simulink model "dbx_control_v0_01"  (R2015a)
settings: Solver=FixedStepDiscrete  SolverMode=SingleTasking  StartTime=0.0  StopTime=10.0  FixedStep=T_ctrl  RelTol=1e-3
values from neighbouring files (symbols this model uses):
  delta_ail_Asim_0 = 0    [FW_init.m]    (also in simple_all.m = single(delta_ail_Asim_0))
  delta_rv_sim_0 = deg2rad(0)    [FW_init.m]    (also in simple_all.m = single(delta_rv_sim_0))
  Euler_0 = zeros(3,1)    [FW_init.m]    (also in simple_all.m = single(Euler_0))
  Euler_0_2 = Euler_0(2)    [FW_init.m]
  FCS_control_mix = inv(B_adim)    [FCS_fw_params.m]
  Flaps_ang_deg = 0    [FCS_fw_params.m]    (also in simple_all.m = single(Flaps_ang_deg))
  Kd_h = 0.05    [FCS_fw_params.m]
  Ki_h = 0.05    [FCS_fw_params.m]
  Ki_p = 0    [FCS_fw_params.m]
  Ki_phi = 0.5    [FCS_fw_params.m]
  Ki_q = 0.01    [FCS_fw_params.m]
  Ki_theta = 0.1    [FCS_fw_params.m]
  Ki_u = 0.03    [FCS_fw_params.m]
  Kp_h = 0.1    [FCS_fw_params.m]
  Kp_p = 0.01    [FCS_fw_params.m]
  Kp_phi = 10    [FCS_fw_params.m]
  Kp_q = 0.07    [FCS_fw_params.m]
  Kp_theta = 3    [FCS_fw_params.m]
  Kp_u = 0.1    [FCS_fw_params.m]
  m = m_OE + m_PL    (= 14.5)    [SetupComplete.m]    (also in simple_all.m = single(m))
  S_w = 0.75    [SetupComplete.m]    (also in simple_all.m = single(S_w))
  T_ctrl = 0.01    [Run_DBX.m]    (also in simple_all.m = double(T_ctrl))
  tau_1_0 = 0.5    [FW_init.m]    (also in simple_all.m = single(tau_1_0))
undefined symbols (not defined in the file or in its folder): Servo_calib
libraries: DBX_model x28, simulink x3
settings Model: ExtModeTrigDuration=5000  TunableVars=Flaps_ang_deg,Kd_h,Ki_h,Ki_p,Ki_phi,Ki_q,Ki_theta,Ki_u,Kp_h,Kp_p,Kp_phi,Kp_q,Kp_theta,Kp_u  TunableVarsStorageClass=Auto,Auto,Auto,Auto,Auto,Auto,Auto,Auto,Auto,Auto,Auto,Auto,Auto,Auto  TunableVarsTypeQualifier=,,,,,,,,,,,,,  Creator=DavidTorres  LastModifiedBy=David
settings DataIOCC: LimitDataPoints=off  SaveOutput=off  SignalLogging=off  DSMLogging=off  VisualizeSimOutput=off  SaveTime=off
settings OptimizationCC: InlineParams=on  UseDivisionForNetSlopeComputation=on  UseSpecifiedMinMax=on  EfficientFloat2IntCast=on  OptimizeModelRefInitCode=on  MaxStackSize=64  SimCompilerOptimization=on
settings DebuggingCC: SaveWithParameterizedLinksMsg=none  IntegerOverflowMsg=error  StrictBusMsg=ErrorOnBusTreatedAsVector  IntegerSaturationMsg=error
settings HardwareCC: ProdLargestAtomicInteger=Long  ProdLargestAtomicFloat=Double  ProdEndianess=LittleEndian  ProdHWDeviceType=ARM Compatible->ARM Cortex  TargetLongLongMode=on  TargetIntDivRoundTo=Zero  TargetEndianess=LittleEndian  TargetHWDeviceType=MATLAB Host  ProdEqTarget=off
settings ModelReferenceCC: ModelReferenceNumInstancesAllowed=Single  ModelReferencePassRootInputsByReference=off
settings RTWCC: SystemTargetFile=ert.tlc  GenCodeOnly=on  TemplateMakefile=ert_default_tmf  Description=Embedded Coder  BuildConfiguration=Faster Runs
settings CodeAppCC: IgnoreCustomStorageClasses=off
settings ERTTargetCC: GenerateSampleERTMain=off  ParMdlRefBuildCompliant=on  CompOptLevelCompliant=on  ConcurrentExecutionCompliant=on  ERTFirstTimeCompliant=on  SupportNonFinite=off  SupportComplex=off  SupportContinuousTime=off  SupportVariableSizeSignals=off  ModelStepFunctionPrototypeControlCompliant=on  CPPClassGenCompliant=on  InlinedParameterPlacement=Hierarchical  ERTCustomFileTemplate=example_file_process.tlc

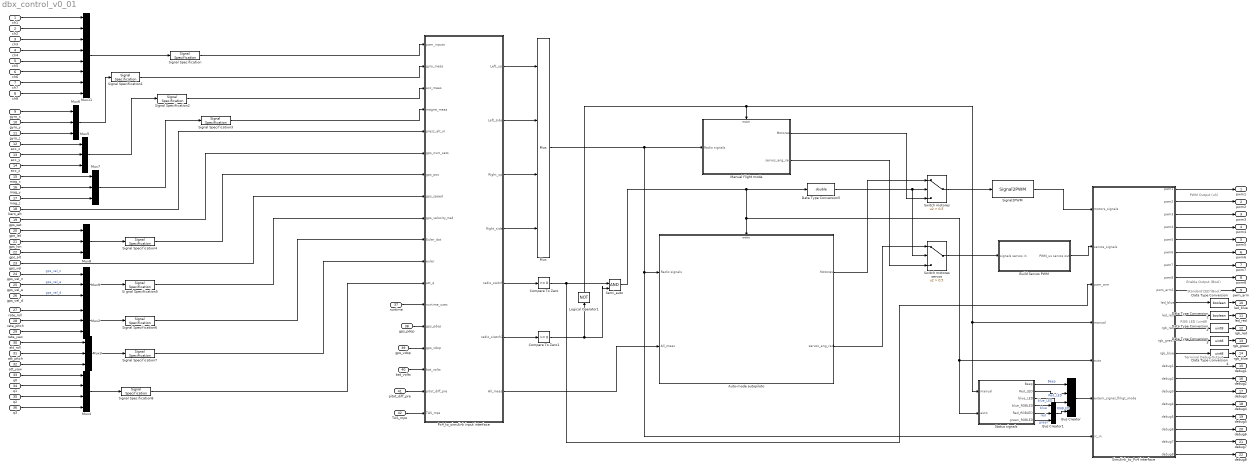
== system dbx_control_v0_01 ==
  note: Terminal Debug Output
  note: RGB LED (uint8)
  note: Standard LED (Bool)
  note: PWM Output (uS)
  note: Enable Output (Bool)
  ch1 : Inport  PortDimensions=[1,1]  SampleTime=T_ctrl
  ch2 : Inport  Port=2  PortDimensions=[1,1]  SampleTime=T_ctrl
  ch3 : Inport  Port=3  PortDimensions=[1,1]  SampleTime=T_ctrl
  ch4 : Inport  Port=4  PortDimensions=[1,1]  SampleTime=T_ctrl
  ch5 : Inport  Port=5  PortDimensions=[1,1]  SampleTime=T_ctrl
  ch6 : Inport  Port=6  PortDimensions=[1,1]  SampleTime=T_ctrl
  ch7 : Inport  Port=7  PortDimensions=[1,1]  SampleTime=T_ctrl
  ch8 : Inport  Port=8  PortDimensions=[1,1]  SampleTime=T_ctrl
  gyro_x : Inport  Port=9  PortDimensions=[1,1]  SampleTime=T_ctrl
  gyro_y : Inport  Port=10  PortDimensions=[1,1]  SampleTime=T_ctrl
  gyro_z : Inport  Port=11  PortDimensions=[1,1]  SampleTime=T_ctrl
  acc_x : Inport  Port=12  PortDimensions=[1,1]  SampleTime=T_ctrl
  acc_y : Inport  Port=13  PortDimensions=[1,1]  SampleTime=T_ctrl
  acc_z : Inport  Port=14  PortDimensions=[1,1]  SampleTime=T_ctrl
  mag_x : Inport  Port=15  PortDimensions=[1,1]  SampleTime=T_ctrl
  mag_y : Inport  Port=16  PortDimensions=[1,1]  SampleTime=T_ctrl
  mag_z : Inport  Port=17  PortDimensions=[1,1]  SampleTime=T_ctrl
  baro_alt : Inport  Port=18  PortDimensions=[1,1]  SampleTime=T_ctrl
  gps_sat : Inport  Port=19  PortDimensions=[1,1]  SampleTime=T_ctrl
  gps_lat : Inport  Port=20  PortDimensions=[1,1]  SampleTime=T_ctrl
  gps_lon : Inport  Port=21  PortDimensions=[1,1]  SampleTime=T_ctrl
  gps_alt : Inport  Port=22  PortDimensions=[1,1]  SampleTime=T_ctrl
  gps_vel : Inport  Port=23  PortDimensions=[1,1]  SampleTime=T_ctrl
  gps_vel_n : Inport  Port=24  PortDimensions=[1,1]  SampleTime=T_ctrl
  gps_vel_e : Inport  Port=25  PortDimensions=[1,1]  SampleTime=T_ctrl
  gps_vel_d : Inport  Port=26  PortDimensions=[1,1]  SampleTime=T_ctrl
  rate_roll : Inport  Port=27  PortDimensions=[1,1]  SampleTime=T_ctrl
  rate_pitch : Inport  Port=28  PortDimensions=[1,1]  SampleTime=T_ctrl
  rate_yaw : Inport  Port=29  PortDimensions=[1,1]  SampleTime=T_ctrl
  att_roll : Inport  Port=30  PortDimensions=[1,1]  SampleTime=T_ctrl
  att_pitch : Inport  Port=31  PortDimensions=[1,1]  SampleTime=T_ctrl
  att_yaw : Inport  Port=32  PortDimensions=[1,1]  SampleTime=T_ctrl
  q0 : Inport  Port=33  PortDimensions=[1,1]  SampleTime=T_ctrl
  q1 : Inport  Port=34  PortDimensions=[1,1]  SampleTime=T_ctrl
  q2 : Inport  Port=35  PortDimensions=[1,1]  SampleTime=T_ctrl
  q3 : Inport  Port=36  PortDimensions=[1,1]  SampleTime=T_ctrl
  runtime : Inport  Port=37  PortDimensions=[1,1]  SampleTime=T_ctrl
  gps_pdop : Inport  Port=38  PortDimensions=[1,1]  SampleTime=T_ctrl
  gps_vdop : Inport  Port=39  PortDimensions=[1,1]  SampleTime=T_ctrl
  bat_volts : Inport  Port=40  PortDimensions=[1,1]  SampleTime=T_ctrl
  pitot_diff_pre : Inport  Port=41  SampleTime=0.01
  TAS_mps : Inport  Port=42  SampleTime=0.01
  Auto-mode autopiloto : Subsystem  TreatAsAtomicUnit=on
  Build Servos PWM : Subsystem  TreatAsAtomicUnit=on
  Bus Creator : BusCreator
  Bus Creator1 : BusCreator  Inputs=3
  Compare To Zero : simulink/Logic and Bit Operations/Compare To Zero  relop=>=  OutDataTypeStr=boolean
  Compare To Zero1 : simulink/Logic and Bit Operations/Compare To Zero  relop=>=  OutDataTypeStr=boolean
  Data Type Conversion : DataTypeConversion  OutDataTypeStr=boolean
  Data Type Conversion1 : DataTypeConversion  OutDataTypeStr=boolean
  Data Type Conversion2 : DataTypeConversion  OutDataTypeStr=uint8
  Data Type Conversion3 : DataTypeConversion  OutDataTypeStr=uint8
  Data Type Conversion4 : DataTypeConversion  OutDataTypeStr=uint8
  Data Type Conversion5 : DataTypeConversion  OutDataTypeStr=double
  Logical Operator1 : Logic  Operator=NOT  IconShape=distinctive  AllPortsSameDT=off  OutDataTypeStr=boolean
  Manual flight mode : Subsystem  TreatAsAtomicUnit=on
  Mux : Mux
  Mux11 : Mux  Inputs=8
  Mux{2..3,5..9} (7 alike) : Mux  Inputs=3
  Mux4 : Mux
  Px4_to_simulink input interface : Subsystem
  Semi_auto : Logic  IconShape=distinctive  AllPortsSameDT=off  OutDataTypeStr=boolean
  Si gnal Specification5 : SignalSpecification  Dimensions=[3,1]
  Signal Specification : SignalSpecification  Dimensions=[8,1]
  Signal Specification{1..4,6..7} (6 alike) : SignalSpecification  Dimensions=[3,1]
  Signal Specification8 : SignalSpecification  Dimensions=[4,1]
  Signal2PWM : DBX_model/Signal2PWM  b=1  d=0  a=1900  c=1100
  Simulink_to_Px4 interface : Subsystem
  Status signals : Subsystem  TreatAsAtomicUnit=on
  Switch motores : Switch  Criteria=u2 > Threshold  Threshold=0.5
  Switch motores servos : Switch  Criteria=u2 > Threshold  Threshold=0.5
  pwm1 : Outport  PortDimensions=[1,1]
  pwm2 : Outport  Port=2  PortDimensions=[1,1]
  pwm3 : Outport  Port=3  PortDimensions=[1,1]
  pwm4 : Outport  Port=4  PortDimensions=[1,1]
  pwm5 : Outport  Port=5  PortDimensions=[1,1]
  pwm6 : Outport  Port=6  PortDimensions=[1,1]
  pwm7 : Outport  Port=7  PortDimensions=[1,1]
  pwm8 : Outport  Port=8  PortDimensions=[1,1]
  pwm_arm : Outport  Port=9  PortDimensions=[1,1]
  led_blue : Outport  Port=10  OutDataTypeStr=boolean  PortDimensions=[1,1]
  led_red : Outport  Port=11  OutDataTypeStr=boolean  PortDimensions=[1,1]
  rgb_red : Outport  Port=12  OutDataTypeStr=uint8  PortDimensions=[1,1]
  rgb_green : Outport  Port=13  OutDataTypeStr=uint8  PortDimensions=[1,1]
  rgb_blue : Outport  Port=14  OutDataTypeStr=uint8  PortDimensions=[1,1]
  debug1 : Outport  Port=15  PortDimensions=[1,1]
  debug2 : Outport  Port=16  PortDimensions=[1,1]
  debug3 : Outport  Port=17  PortDimensions=[1,1]
  debug4 : Outport  Port=18  PortDimensions=[1,1]
  debug5 : Outport  Port=19  PortDimensions=[1,1]
  debug6 : Outport  Port=20  PortDimensions=[1,1]
  debug7 : Outport  Port=21  PortDimensions=[1,1]
  debug8 : Outport  Port=22  PortDimensions=[1,1]
  wires:
  Switch motores/1 -> Signal2PWM/1
  Switch motores servos/1 -> Build Servos PWM/1(signals servos in)
  Status signals/1(Beep) -> Bus Creator/1  "Beep"
  Status signals/2(Red_LED) -> Bus Creator/2  "Red_LED"
  Status signals/3(blue_LED) -> Bus Creator/3  "blue_LED"
  Status signals/4(blue_RGBLED) -> Bus Creator1/1  "blue"
  Status signals/5(Red_RGBLED) -> Bus Creator1/2  "red"
  Status signals/6(green_RGBLED) -> Bus Creator1/3  "green"
  Bus Creator1/1 -> Bus Creator/4  "RGBLED"
  Simulink_to_Px4 interface/1(pwm1) -> pwm1/1
  Simulink_to_Px4 interface/2(pwm2) -> pwm2/1
  Simulink_to_Px4 interface/3(pwm3) -> pwm3/1
  Simulink_to_Px4 interface/4(pwm4) -> pwm4/1
  Simulink_to_Px4 interface/5(pwm5) -> pwm5/1
  Simulink_to_Px4 interface/6(pwm6) -> pwm6/1
  Simulink_to_Px4 interface/7(pwm7) -> pwm7/1
  Simulink_to_Px4 interface/8(pwm8) -> pwm8/1
  Simulink_to_Px4 interface/10(led_blue) -> Data Type Conversion/1
  Simulink_to_Px4 interface/11(led_red) -> Data Type Conversion1/1
  Simulink_to_Px4 interface/15(debug1) -> debug1/1
  Simulink_to_Px4 interface/17(debug3) -> debug3/1
  Simulink_to_Px4 interface/18(debug4) -> debug4/1
  Simulink_to_Px4 interface/9(pwm_arm1) -> pwm_arm/1
  Simulink_to_Px4 interface/12(rgb_red) -> Data Type Conversion2/1
  Simulink_to_Px4 interface/13(rgb_green) -> Data Type Conversion3/1
  Simulink_to_Px4 interface/14(rgb_blue) -> Data Type Conversion4/1
  Simulink_to_Px4 interface/20(debug6) -> debug6/1
  Simulink_to_Px4 interface/21(debug7) -> debug7/1
  Simulink_to_Px4 interface/22(debug8) -> debug8/1
  Simulink_to_Px4 interface/19(debug5) -> debug5/1
  Data Type Conversion/1 -> led_blue/1
  Data Type Conversion1/1 -> led_red/1
  Data Type Conversion2/1 -> rgb_red/1
  Data Type Conversion3/1 -> rgb_green/1
  Data Type Conversion4/1 -> rgb_blue/1
  Simulink_to_Px4 interface/16(debug2) -> debug2/1
  Signal2PWM/1 -> Simulink_to_Px4 interface/1(motors_signals)
  Build Servos PWM/1(PWM_us servos out) -> Simulink_to_Px4 interface/2(servos_signals)
  Bus Creator/1 -> Simulink_to_Px4 interface/6(extern_signal_flihgt_mode)
  baro_alt/1 -> Px4_to_simulink input interface/5(press_alt_m)
  gyro_z/1 -> Mux6/3
  gyro_y/1 -> Mux6/2
  gyro_x/1 -> Mux6/1
  acc_z/1 -> Mux5/3
  acc_y/1 -> Mux5/2
  acc_x/1 -> Mux5/1
  mag_x/1 -> Mux7/1
  mag_y/1 -> Mux7/2
  mag_z/1 -> Mux7/3
  ch1/1 -> Mux11/1
  ch2/1 -> Mux11/2
  ch3/1 -> Mux11/3
  ch4/1 -> Mux11/4
  ch5/1 -> Mux11/5
  ch6/1 -> Mux11/6
  runtime/1 -> Px4_to_simulink input interface/13(runtime_usec)
  ch7/1 -> Mux11/7
  ch8/1 -> Mux11/8
  att_roll/1 -> Mux3/1
  att_pitch/1 -> Mux3/2
  att_yaw/1 -> Mux3/3
  q0/1 -> Mux4/1
  q1/1 -> Mux4/2
  q2/1 -> Mux4/3
  q3/1 -> Mux4/4
  rate_roll/1 -> Mux2/1
  rate_pitch/1 -> Mux2/2
  rate_yaw/1 -> Mux2/3
  gps_vel_n/1 -> Mux9/1  "gps_vel_n"
  gps_vel_e/1 -> Mux9/2  "gps_vel_e"
  gps_vel_d/1 -> Mux9/3  "gps_vel_d"
  gps_lat/1 -> Mux8/1
  gps_lon/1 -> Mux8/2
  gps_alt/1 -> Mux8/3
  gps_vel/1 -> Px4_to_simulink input interface/8(gps_speed)
  gps_sat/1 -> Px4_to_simulink input interface/6(gps_num_sats)
  Mux2/1 -> Signal Specification6/1
  Mux3/1 -> Signal Specification7/1
  Mux4/1 -> Signal Specification8/1
  Mux5/1 -> Signal Specification2/1
  Mux6/1 -> Signal Specification1/1
  Mux8/1 -> Signal Specification4/1
  Mux7/1 -> Signal Specification3/1
  Mux11/1 -> Signal Specification/1
  Mux9/1 -> Si gnal Specification5/1
  gps_pdop/1 -> Px4_to_simulink input interface/14(gps_pdop)
  gps_vdop/1 -> Px4_to_simulink input interface/15(gps_vdop)
  bat_volts/1 -> Px4_to_simulink input interface/16(bat_volts)
  Signal Specification/1 -> Px4_to_simulink input interface/1(pwm_inputs)
  Signal Specification1/1 -> Px4_to_simulink input interface/2(gyro_meas)
  Signal Specification2/1 -> Px4_to_simulink input interface/3(acc_meas)
  Signal Specification3/1 -> Px4_to_simulink input interface/4(magne_meas)
  Signal Specification4/1 -> Px4_to_simulink input interface/7(gps_pos)
  Si gnal Specification5/1 -> Px4_to_simulink input interface/9(gps_velocity_ned)
  Signal Specification6/1 -> Px4_to_simulink input interface/10(Euler_dot)
  Signal Specification7/1 -> Px4_to_simulink input interface/11(euler)
  Signal Specification8/1 -> Px4_to_simulink input interface/12(att_q)
  pitot_diff_pre/1 -> Px4_to_simulink input interface/17(pitot_diff_pre)
  Px4_to_simulink input interface/5(radio_switch) -> Compare To Zero/1
  Px4_to_simulink input interface/6(radio_siwtch2) -> Compare To Zero1/1
  Compare To Zero/1 -> Semi_auto/1, Simulink_to_Px4 interface/3(pwm_arm)
  Compare To Zero1/1 -> Logical Operator1/1, Semi_auto/2
  Logical Operator1/1 -> Simulink_to_Px4 interface/4(manual), Status signals/1(manual), Manual flight mode/Enable
  Manual flight mode/1(Motores) -> Switch motores/3
  Manual flight mode/2(servos_ang_rad) -> Switch motores servos/3
  Auto-mode autopiloto/1(Motores) -> Switch motores/1
  Auto-mode autopiloto/2(servos_ang_rad) -> Switch motores servos/1
  Semi_auto/1 -> Data Type Conversion5/1, Simulink_to_Px4 interface/5(auto), Status signals/2(auto), Auto-mode autopiloto/Enable
  Data Type Conversion5/1 -> Switch motores servos/2, Switch motores/2
  Px4_to_simulink input interface/4(Right_side) -> Mux/4
  Px4_to_simulink input interface/3(Right_up) -> Mux/3
  Px4_to_simulink input interface/2(Left_side) -> Mux/2
  Px4_to_simulink input interface/1(Left_up) -> Mux/1
  Px4_to_simulink input interface/7(All_meas) -> Auto-mode autopiloto/2(All_meas)
  Mux/1 -> Simulink_to_Px4 interface/7(rc_in), Auto-mode autopiloto/1(Radio signals), Manual flight mode/1(Radio signals)
  TAS_mps/1 -> Px4_to_simulink input interface/18(TAS_mps)

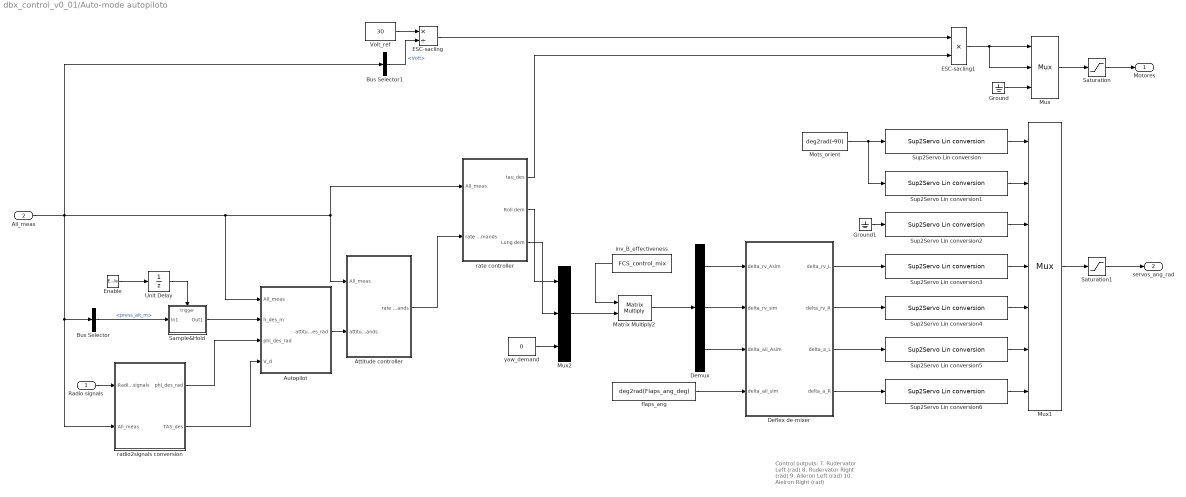
== system dbx_control_v0_01/Auto-mode autopiloto ==
  note: Control outputs:
      |
      |
      | 7. Rudervator Left (rad)
      | 8. Rudervator Right (rad)
      | 9. Aileron Left (rad)
      | 10. Aielron Right (rad)
  Radio signals : Inport
  All_meas : Inport  Port=2
  Enable : EnablePort  ShowOutputPort=on
  Attitude controller : Subsystem
  Autopilot : Subsystem
  Bus Selector : BusSelector  OutputSignals=Meas.press_alt_m
  Bus Selector1 : BusSelector  OutputSignals=Meas.Volt
  Deflex de-mixer : Subsystem  TreatAsAtomicUnit=on
  Demux : Demux  Outputs=3
  ESC-sacling : Product  Inputs=*/
  ESC-sacling1 : Product  Inputs=**
  Ground : Ground
  Ground1 : Ground
  Matrix Multiply2 : Product  Multiplication=Matrix(*)
  Mots_orient : Constant  Value=deg2rad(-90)
  Mux : Mux  Inputs=3
  Mux1 : Mux  Inputs=7
  Mux2 : Mux  Inputs=3
  Sample&Hold : Subsystem  TreatAsAtomicUnit=on
  Saturation : Saturate  UpperLimit=1  LowerLimit=0
  Saturation1 : Saturate  UpperLimit=deg2rad(90)  LowerLimit=-deg2rad(90)
  Sup2Servo Lin conversion : DBX_model/Sup2Servo Lin conversion  Gain=Servo_calib.Servo1.Pendiente_Sup_Servo  Bias=Servo_calib.Servo1.Sup_rad_0
  Sup2Servo Lin conversion1 : DBX_model/Sup2Servo Lin conversion  Gain=Servo_calib.Servo2.Pendiente_Sup_Servo  Bias=Servo_calib.Servo2.Sup_rad_0
  Sup2Servo Lin conversion2 : DBX_model/Sup2Servo Lin conversion  Gain=Servo_calib.Servo3.Pendiente_Sup_Servo  Bias=Servo_calib.Servo3.Sup_rad_0
  Sup2Servo Lin conversion3 : DBX_model/Sup2Servo Lin conversion  Gain=Servo_calib.Servo4.Pendiente_Sup_Servo  Bias=Servo_calib.Servo4.Sup_rad_0
  Sup2Servo Lin conversion4 : DBX_model/Sup2Servo Lin conversion  Gain=Servo_calib.Servo5.Pendiente_Sup_Servo  Bias=Servo_calib.Servo5.Sup_rad_0
  Sup2Servo Lin conversion5 : DBX_model/Sup2Servo Lin conversion  Gain=Servo_calib.Servo6.Pendiente_Sup_Servo  Bias=Servo_calib.Servo6.Sup_rad_0
  Sup2Servo Lin conversion6 : DBX_model/Sup2Servo Lin conversion  Gain=Servo_calib.Servo7.Pendiente_Sup_Servo  Bias=Servo_calib.Servo7.Sup_rad_0
  Unit Delay : UnitDelay  SampleTime=-1
  Volt_ref : Constant  Value=30
  flaps_ang : Constant  Value=deg2rad(Flaps_ang_deg)
  inv_B_effectiveness : Constant  Value=FCS_control_mix
  radio2signals conversion : Subsystem
  rate controller : Subsystem
  yaw_demand : Constant  Value=0
  Motores : Outport
  servos_ang_rad : Outport  Port=2
  wires:
  Mux/1 -> Saturation/1
  Saturation/1 -> Motores/1
  Ground/1 -> Mux/3
  Mux1/1 -> Saturation1/1
  Saturation1/1 -> servos_ang_rad/1
  Ground1/1 -> Sup2Servo Lin conversion2/1
  Sup2Servo Lin conversion/1 -> Mux1/1
  Sup2Servo Lin conversion1/1 -> Mux1/2
  Sup2Servo Lin conversion2/1 -> Mux1/3
  Mots_orient/1 -> Sup2Servo Lin conversion1/1, Sup2Servo Lin conversion/1
  Deflex de-mixer/4(delta_a_R) -> Sup2Servo Lin conversion6/1
  Deflex de-mixer/3(delta_a_L) -> Sup2Servo Lin conversion5/1
  Deflex de-mixer/2(delta_rv_R) -> Sup2Servo Lin conversion4/1
  Deflex de-mixer/1(delta_rv_L) -> Sup2Servo Lin conversion3/1
  flaps_ang/1 -> Deflex de-mixer/4(delta_ail_sim)
  Demux/1 -> Deflex de-mixer/1(delta_rv_Asim)
  Demux/2 -> Deflex de-mixer/2(delta_rv_sim)
  Demux/3 -> Deflex de-mixer/3(delta_ail_Asim)
  Sup2Servo Lin conversion3/1 -> Mux1/4
  Sup2Servo Lin conversion4/1 -> Mux1/5
  Sup2Servo Lin conversion5/1 -> Mux1/6
  Sup2Servo Lin conversion6/1 -> Mux1/7
  Enable/1 -> Unit Delay/1
  Unit Delay/1 -> Sample&Hold/Trigger
  Volt_ref/1 -> ESC-sacling/1
  Bus Selector1/1 -> ESC-sacling/2  "<Volt>"
  ESC-sacling1/1 -> Mux/2, Mux/1
  ESC-sacling/1 -> ESC-sacling1/1
  rate controller/1(tau_des) -> ESC-sacling1/2
  Bus Selector/1 -> Sample&Hold/1(In1)  "<press_alt_m>"
  Sample&Hold/1(Out1) -> Autopilot/2(h_des_m)
  Autopilot/1(attitude_des_rad) -> Attitude controller/2(attitude demands)
  Attitude controller/1(rate demands) -> rate controller/2(rate demands)
  Radio signals/1 -> radio2signals conversion/1(Radio_signals)
  radio2signals conversion/1(phi_des_rad) -> Autopilot/3(phi_des_rad)
  radio2signals conversion/2(TAS_des) -> Autopilot/4(V_d)
  All_meas/1 -> Bus Selector/1, radio2signals conversion/2(All_meas), Autopilot/1(All_meas), Attitude controller/1(All_meas), rate controller/1(All_meas), Bus Selector1/1
  rate controller/2(Roll dem) -> Mux2/1
  rate controller/3(Long dem) -> Mux2/2
  yaw_demand/1 -> Mux2/3
  inv_B_effectiveness/1 -> Matrix Multiply2/1
  Mux2/1 -> Matrix Multiply2/2
  Matrix Multiply2/1 -> Demux/1

== system dbx_control_v0_01/Build Servos PWM ==
  note: Estos 4 ultimos significa que
      | los ejes de los servos deben
      | apuntar el la direccion +y
  note: Control input
      | Rango
      | Direccion rot/Dir servos
      | Rango del servo
      |
      | eta_1 (rad) (Pan arm 1)
      | -90,90
      | -1
      | 180
      |
      | eta_2 (rad) (Pan arm 2
      | -90,90
      | -1
      | 180
      |
      | eta_3 (rad) (Pan arm 3)
      | -90,90
      | 1
      | 180
      |
      | Rudervator Left (rad)
      | -90,90
      | 1
      | 180
      |
      | Rudervator Right (rad)
      | -90,90
      | 1
      | 180
      |
      | Aileron Left (rad)
      | -90,90
      | 1
      | 180
      |
      | Aielron Right (rad)
      | -90,90
      | 1
      | 180
  signals servos in : Inport
  Demux : Demux  Outputs=7
  Mux : Mux  Inputs=7
  Signal2PWM{,1..6} (7 alike) : DBX_model/Signal2PWM  b=deg2rad(90)  d=-deg2rad(90)  a=1900  c=1100
  PWM_us servos out : Outport
  wires:
  Mux/1 -> PWM_us servos out/1
  signals servos in/1 -> Demux/1
  Demux/6 -> Signal2PWM5/1
  Demux/5 -> Signal2PWM4/1
  Demux/4 -> Signal2PWM3/1
  Demux/3 -> Signal2PWM2/1
  Demux/2 -> Signal2PWM1/1
  Demux/1 -> Signal2PWM/1
  Signal2PWM/1 -> Mux/1
  Signal2PWM1/1 -> Mux/2
  Signal2PWM3/1 -> Mux/4
  Signal2PWM4/1 -> Mux/5
  Signal2PWM2/1 -> Mux/3
  Signal2PWM5/1 -> Mux/6
  Demux/7 -> Signal2PWM6/1
  Signal2PWM6/1 -> Mux/7

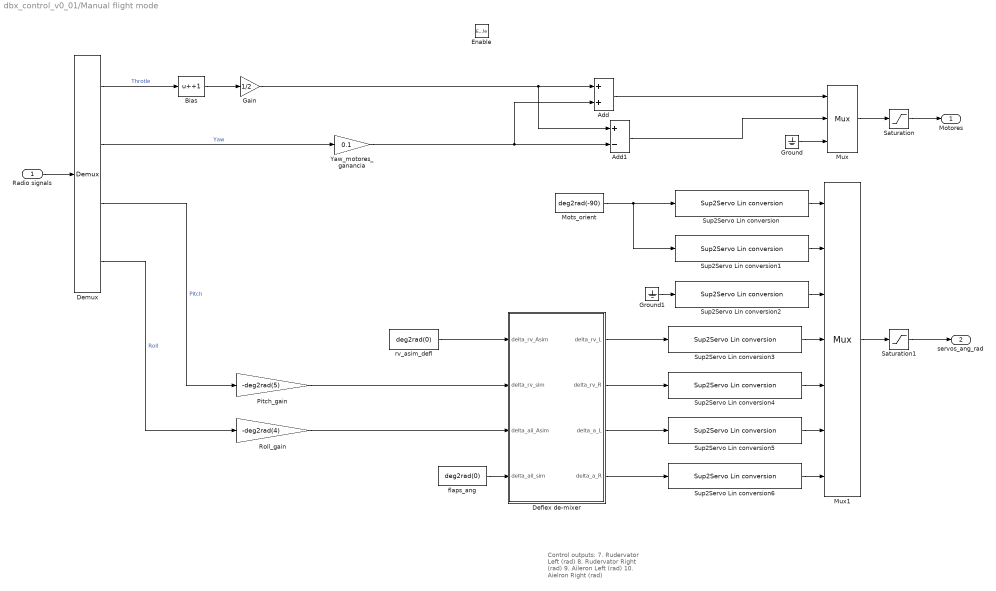
== system dbx_control_v0_01/Manual flight mode ==
  note: Control outputs:
      |
      |
      | 7. Rudervator Left (rad)
      | 8. Rudervator Right (rad)
      | 9. Aileron Left (rad)
      | 10. Aielron Right (rad)
  Radio signals : Inport
  Enable : EnablePort
  Add : Sum
  Add1 : Sum  Inputs=+-
  Bias : Bias  Bias=+1
  Deflex de-mixer : Subsystem  TreatAsAtomicUnit=on
  Demux : Demux
  Gain : Gain  Gain=1/2
  Ground : Ground
  Ground1 : Ground
  Mots_orient : Constant  Value=deg2rad(-90)
  Mux : Mux  Inputs=3
  Mux1 : Mux  Inputs=7
  Pitch_gain : Gain  Gain=-deg2rad(5)
  Roll_gain : Gain  Gain=-deg2rad(4)
  Saturation : Saturate  UpperLimit=1  LowerLimit=0
  Saturation1 : Saturate  UpperLimit=deg2rad(90)  LowerLimit=-deg2rad(90)
  Sup2Servo Lin conversion : DBX_model/Sup2Servo Lin conversion  Gain=Servo_calib.Servo1.Pendiente_Sup_Servo  Bias=Servo_calib.Servo1.Sup_rad_0
  Sup2Servo Lin conversion1 : DBX_model/Sup2Servo Lin conversion  Gain=Servo_calib.Servo2.Pendiente_Sup_Servo  Bias=Servo_calib.Servo2.Sup_rad_0
  Sup2Servo Lin conversion2 : DBX_model/Sup2Servo Lin conversion  Gain=Servo_calib.Servo3.Pendiente_Sup_Servo  Bias=Servo_calib.Servo3.Sup_rad_0
  Sup2Servo Lin conversion3 : DBX_model/Sup2Servo Lin conversion  Gain=Servo_calib.Servo4.Pendiente_Sup_Servo  Bias=Servo_calib.Servo4.Sup_rad_0
  Sup2Servo Lin conversion4 : DBX_model/Sup2Servo Lin conversion  Gain=Servo_calib.Servo5.Pendiente_Sup_Servo  Bias=Servo_calib.Servo5.Sup_rad_0
  Sup2Servo Lin conversion5 : DBX_model/Sup2Servo Lin conversion  Gain=Servo_calib.Servo6.Pendiente_Sup_Servo  Bias=Servo_calib.Servo6.Sup_rad_0
  Sup2Servo Lin conversion6 : DBX_model/Sup2Servo Lin conversion  Gain=Servo_calib.Servo7.Pendiente_Sup_Servo  Bias=Servo_calib.Servo7.Sup_rad_0
  Yaw_motores_ganancia : Gain  Gain=0.1
  flaps_ang : Constant  Value=deg2rad(0)
  rv_asim_defl : Constant  Value=deg2rad(0)
  Motores : Outport
  servos_ang_rad : Outport  Port=2
  wires:
  Radio signals/1 -> Demux/1
  Mux/1 -> Saturation/1
  Saturation/1 -> Motores/1
  Demux/1 -> Bias/1  "Throtle"
  Ground/1 -> Mux/3
  Bias/1 -> Gain/1
  Gain/1 -> Add1/1, Add/1
  Demux/2 -> Yaw_motores_ganancia/1  "Yaw"
  Add/1 -> Mux/1
  Yaw_motores_ganancia/1 -> Add1/2, Add/2
  Add1/1 -> Mux/2
  Demux/3 -> Pitch_gain/1  "Pitch"
  Demux/4 -> Roll_gain/1  "Roll"
  Mux1/1 -> Saturation1/1
  Saturation1/1 -> servos_ang_rad/1
  Ground1/1 -> Sup2Servo Lin conversion2/1
  Sup2Servo Lin conversion/1 -> Mux1/1
  Sup2Servo Lin conversion1/1 -> Mux1/2
  Sup2Servo Lin conversion2/1 -> Mux1/3
  Mots_orient/1 -> Sup2Servo Lin conversion1/1, Sup2Servo Lin conversion/1
  Deflex de-mixer/4(delta_a_R) -> Sup2Servo Lin conversion6/1
  Deflex de-mixer/3(delta_a_L) -> Sup2Servo Lin conversion5/1
  Deflex de-mixer/2(delta_rv_R) -> Sup2Servo Lin conversion4/1
  Deflex de-mixer/1(delta_rv_L) -> Sup2Servo Lin conversion3/1
  flaps_ang/1 -> Deflex de-mixer/4(delta_ail_sim)
  rv_asim_defl/1 -> Deflex de-mixer/1(delta_rv_Asim)
  Pitch_gain/1 -> Deflex de-mixer/2(delta_rv_sim)
  Roll_gain/1 -> Deflex de-mixer/3(delta_ail_Asim)
  Sup2Servo Lin conversion3/1 -> Mux1/4
  Sup2Servo Lin conversion4/1 -> Mux1/5
  Sup2Servo Lin conversion5/1 -> Mux1/6
  Sup2Servo Lin conversion6/1 -> Mux1/7

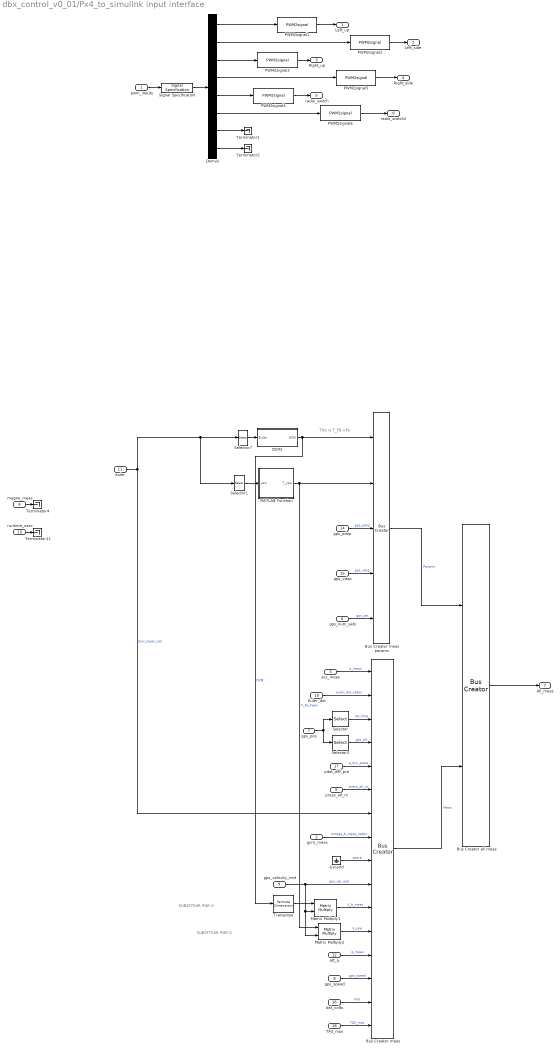
== system dbx_control_v0_01/Px4_to_simulink input interface ==
  note: SUBSTITUIR POR 0
  note: This is T_Fb->Fe
  note: SUBSTITUIR POR 0
  pwm_inputs : Inport  PortDimensions=8  SampleTime=T_ctrl
  gyro_meas : Inport  Port=2  PortDimensions=3  SampleTime=T_ctrl
  acc_meas : Inport  Port=3  PortDimensions=3  SampleTime=T_ctrl
  magne_meas : Inport  Port=4  PortDimensions=3  SampleTime=T_ctrl
  press_alt_m : Inport  Port=5  PortDimensions=1  SampleTime=T_ctrl
  gps_num_sats : Inport  Port=6  PortDimensions=1  SampleTime=T_ctrl
  gps_pos : Inport  Port=7  PortDimensions=3  SampleTime=T_ctrl
  gps_speed : Inport  Port=8  PortDimensions=1  SampleTime=T_ctrl
  gps_velocity_ned : Inport  Port=9  PortDimensions=3  SampleTime=T_ctrl
  Euler_dot : Inport  Port=10  PortDimensions=3  SampleTime=T_ctrl
  euler : Inport  Port=11  PortDimensions=3  SampleTime=T_ctrl
  att_q : Inport  Port=12  PortDimensions=4  SampleTime=T_ctrl
  runtime_usec : Inport  Port=13  PortDimensions=1  SampleTime=T_ctrl
  gps_pdop : Inport  Port=14  PortDimensions=1  SampleTime=T_ctrl
  gps_vdop : Inport  Port=15  PortDimensions=1  SampleTime=T_ctrl
  bat_volts : Inport  Port=16  PortDimensions=1  SampleTime=T_ctrl
  pitot_diff_pre : Inport  Port=17  SampleTime=0.01
  TAS_mps : Inport  Port=18  SampleTime=0.01
  Bus Creator all meas : BusCreator  Inputs=2
  Bus Creator meas : BusCreator  Inputs=16
  Bus Creator meas params : BusCreator  Inputs=5
  DCM1 : Subsystem  TreatAsAtomicUnit=on
  Demux : Demux  Outputs=8
  Ground : Ground
  MATLAB Function : MATLAB Function  TreatAsAtomicUnit=on
  Matrix Multiply1 : Product  Multiplication=Matrix(*)
  Matrix Multiply2 : Product  Multiplication=Matrix(*)
  PWM2signal{1..6} (6 alike) : DBX_model/PWM2signal  c=2000  a=1000  d=1  b=-1
  Selector : Selector  InputPortWidth=3  Indices=[1,2]
  Selector1 : Selector  InputPortWidth=3  Indices=3
  Selector2 : Selector  InputPortWidth=3  Indices=3
  Selector7 : Selector  InputPortWidth=3  Indices=[3 2 1]
  Signal Specification : SignalSpecification  Dimensions=8
  Terminator{1..2,4,11} (4 alike) : Terminator
  Transpose : PermuteDimensions
  Left_up : Outport
  Left_side : Outport  Port=2
  Right_up : Outport  Port=3
  Right_side : Outport  Port=4
  radio_switch : Outport  Port=5
  radio_siwtch2 : Outport  Port=6
  All_meas : Outport  Port=7
  wires:
  PWM2signal1/1 -> Left_up/1
  PWM2signal2/1 -> Left_side/1
  PWM2signal3/1 -> Right_up/1
  PWM2signal5/1 -> Right_side/1
  Bus Creator all meas/1 -> All_meas/1
  PWM2signal4/1 -> radio_switch/1
  att_q/1 -> Bus Creator meas/13  "q_meas"
  euler/1 -> Bus Creator meas/7, Selector1/1, Selector7/1  "Eulr_meas_rad"
  Euler_dot/1 -> Bus Creator meas/2  "euler_dot_radps"
  bat_volts/1 -> Bus Creator meas/15  "Volt"
  Bus Creator meas/1 -> Bus Creator all meas/2  "Meas"
  Bus Creator meas params/1 -> Bus Creator all meas/1  "Params"
  DCM1/1(DCM) -> Transpose/1, Bus Creator meas params/1  "DCM"
  acc_meas/1 -> Bus Creator meas/1  "a_meas"
  gps_pdop/1 -> Bus Creator meas params/3  "gps_pdop"
  gps_num_sats/1 -> Bus Creator meas params/5  "gps_sat"
  gps_vdop/1 -> Bus Creator meas params/4  "gps_vdop"
  Selector7/1 -> DCM1/1(Euler)
  Selector1/1 -> MATLAB Function/1(yaw)
  MATLAB Function/1(T_yaw) -> Matrix Multiply2/1, Bus Creator meas params/2  "T_Fe_Fyaw"
  Demux/1 -> PWM2signal1/1
  Demux/2 -> PWM2signal2/1
  Demux/3 -> PWM2signal3/1
  Demux/4 -> PWM2signal5/1
  Demux/5 -> PWM2signal4/1
  pwm_inputs/1 -> Signal Specification/1
  Demux/6 -> PWM2signal6/1
  Demux/7 -> Terminator1/1
  Demux/8 -> Terminator2/1
  gyro_meas/1 -> Bus Creator meas/8  "omega_b_meas_radps"
  magne_meas/1 -> Terminator4/1
  press_alt_m/1 -> Bus Creator meas/6  "press_alt_m"
  gps_pos/1 -> Selector2/1, Selector/1
  gps_speed/1 -> Bus Creator meas/14  "gps_speed"
  gps_velocity_ned/1 -> Bus Creator meas/10, Matrix Multiply2/2, Matrix Multiply1/2  "gps_vel_ned"
  runtime_usec/1 -> Terminator11/1
  Signal Specification/1 -> Demux/1
  PWM2signal6/1 -> radio_siwtch2/1
  pitot_diff_pre/1 -> Bus Creator meas/5  "q_dyn_press"
  Selector/1 -> Bus Creator meas/3  "lat_long"
  Selector2/1 -> Bus Creator meas/4  "gps_alt"
  TAS_mps/1 -> Bus Creator meas/16  "TAS_mps"
  Transpose/1 -> Matrix Multiply1/1
  Matrix Multiply1/1 -> Bus Creator meas/11  "V_b_meas"
  Matrix Multiply2/1 -> Bus Creator meas/12  "V_yaw"
  Ground/1 -> Bus Creator meas/9  "spare"

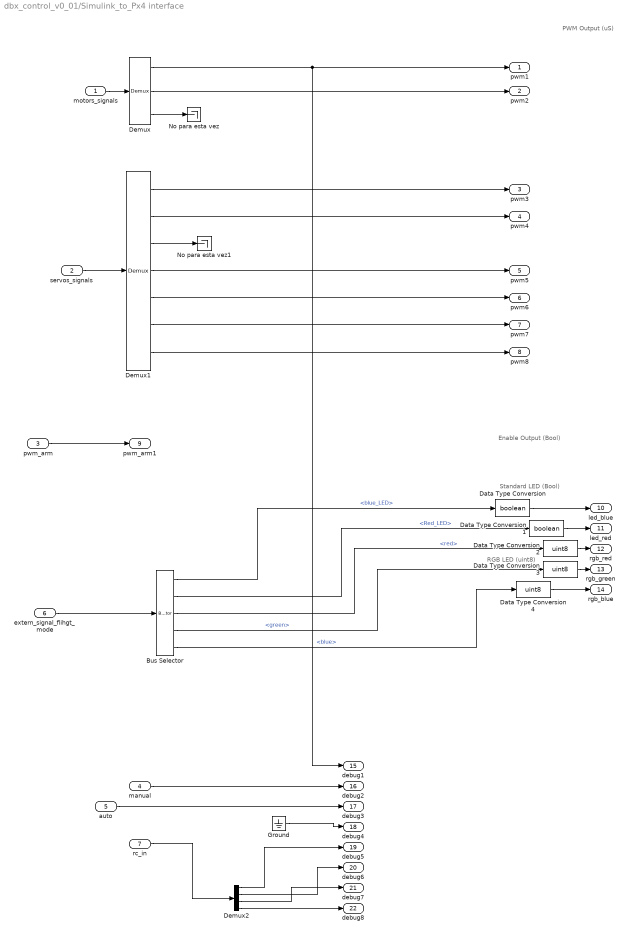
== system dbx_control_v0_01/Simulink_to_Px4 interface ==
  note: RGB LED (uint8)
  note: Standard LED (Bool)
  note: PWM Output (uS)
  note: Enable Output (Bool)
  motors_signals : Inport
  servos_signals : Inport  Port=2
  pwm_arm : Inport  Port=3
  manual : Inport  Port=4
  auto : Inport  Port=5
  extern_signal_flihgt_mode : Inport  Port=6
  rc_in : Inport  Port=7
  Bus Selector : BusSelector  OutputSignals=blue_LED,Red_LED,RGBLED.red,RGBLED.green,RGBLED.blue
  Data Type Conversion : DataTypeConversion  OutDataTypeStr=boolean
  Data Type Conversion1 : DataTypeConversion  OutDataTypeStr=boolean
  Data Type Conversion2 : DataTypeConversion  OutDataTypeStr=uint8
  Data Type Conversion3 : DataTypeConversion  OutDataTypeStr=uint8
  Data Type Conversion4 : DataTypeConversion  OutDataTypeStr=uint8
  Demux : Demux  Outputs=3
  Demux1 : Demux  Outputs=7
  Demux2 : Demux
  Ground : Ground
  No para esta vez : Terminator
  No para esta vez1 : Terminator
  pwm1 : Outport  PortDimensions=1  SampleTime=T_ctrl
  pwm2 : Outport  Port=2  PortDimensions=1  SampleTime=T_ctrl
  pwm3 : Outport  Port=3  PortDimensions=1  SampleTime=T_ctrl
  pwm4 : Outport  Port=4  PortDimensions=1  SampleTime=T_ctrl
  pwm5 : Outport  Port=5  PortDimensions=1  SampleTime=T_ctrl
  pwm6 : Outport  Port=6  PortDimensions=1  SampleTime=T_ctrl
  pwm7 : Outport  Port=7  PortDimensions=1  SampleTime=T_ctrl
  pwm8 : Outport  Port=8  PortDimensions=1  SampleTime=T_ctrl
  pwm_arm1 : Outport  Port=9  PortDimensions=1  SampleTime=T_ctrl
  led_blue : Outport  Port=10  OutDataTypeStr=boolean  PortDimensions=1  SampleTime=T_ctrl
  led_red : Outport  Port=11  OutDataTypeStr=boolean  PortDimensions=1  SampleTime=T_ctrl
  rgb_red : Outport  Port=12  OutDataTypeStr=uint8  PortDimensions=1  SampleTime=T_ctrl
  rgb_green : Outport  Port=13  OutDataTypeStr=uint8  PortDimensions=1  SampleTime=T_ctrl
  rgb_blue : Outport  Port=14  OutDataTypeStr=uint8  PortDimensions=1  SampleTime=T_ctrl
  debug1 : Outport  Port=15  PortDimensions=1  SampleTime=T_ctrl
  debug2 : Outport  Port=16  PortDimensions=1  SampleTime=T_ctrl
  debug3 : Outport  Port=17  PortDimensions=1  SampleTime=T_ctrl
  debug4 : Outport  Port=18  PortDimensions=1  SampleTime=T_ctrl
  debug5 : Outport  Port=19  PortDimensions=1  SampleTime=T_ctrl
  debug6 : Outport  Port=20  PortDimensions=1  SampleTime=T_ctrl
  debug7 : Outport  Port=21  PortDimensions=1  SampleTime=T_ctrl
  debug8 : Outport  Port=22  PortDimensions=1  SampleTime=T_ctrl
  wires:
  extern_signal_flihgt_mode/1 -> Bus Selector/1
  Bus Selector/2 -> Data Type Conversion1/1  "<Red_LED>"
  pwm_arm/1 -> pwm_arm1/1
  Bus Selector/3 -> Data Type Conversion2/1  "<red>"
  Bus Selector/4 -> Data Type Conversion3/1  "<green>"
  Bus Selector/5 -> Data Type Conversion4/1  "<blue>"
  Data Type Conversion/1 -> led_blue/1
  Data Type Conversion1/1 -> led_red/1
  Data Type Conversion2/1 -> rgb_red/1
  Data Type Conversion3/1 -> rgb_green/1
  Data Type Conversion4/1 -> rgb_blue/1
  Bus Selector/1 -> Data Type Conversion/1  "<blue_LED>"
  motors_signals/1 -> Demux/1
  Demux/1 -> debug1/1, pwm1/1
  Demux/2 -> pwm2/1
  Demux/3 -> No para esta vez/1
  servos_signals/1 -> Demux1/1
  Demux1/1 -> pwm3/1
  Demux1/2 -> pwm4/1
  Demux1/3 -> No para esta vez1/1
  Demux1/4 -> pwm5/1
  Demux1/5 -> pwm6/1
  Demux1/6 -> pwm7/1
  Demux1/7 -> pwm8/1
  rc_in/1 -> Demux2/1
  manual/1 -> debug2/1
  auto/1 -> debug3/1
  Demux2/4 -> debug8/1
  Demux2/3 -> debug7/1
  Demux2/2 -> debug6/1
  Demux2/1 -> debug5/1
  Ground/1 -> debug4/1

== system dbx_control_v0_01/Status signals ==
  manual : Inport
  auto : Inport  Port=2
  Ground : Ground
  Ground1 : Ground
  Beep : Outport
  Red_LED : Outport  Port=2
  blue_LED : Outport  Port=3
  blue_RGBLED : Outport  Port=4
  Red_RGBLED : Outport  Port=5
  green_RGBLED : Outport  Port=6
  wires:
  Ground/1 -> blue_RGBLED/1, Red_RGBLED/1, green_RGBLED/1
  Ground1/1 -> Beep/1
  manual/1 -> Red_LED/1
  auto/1 -> blue_LED/1

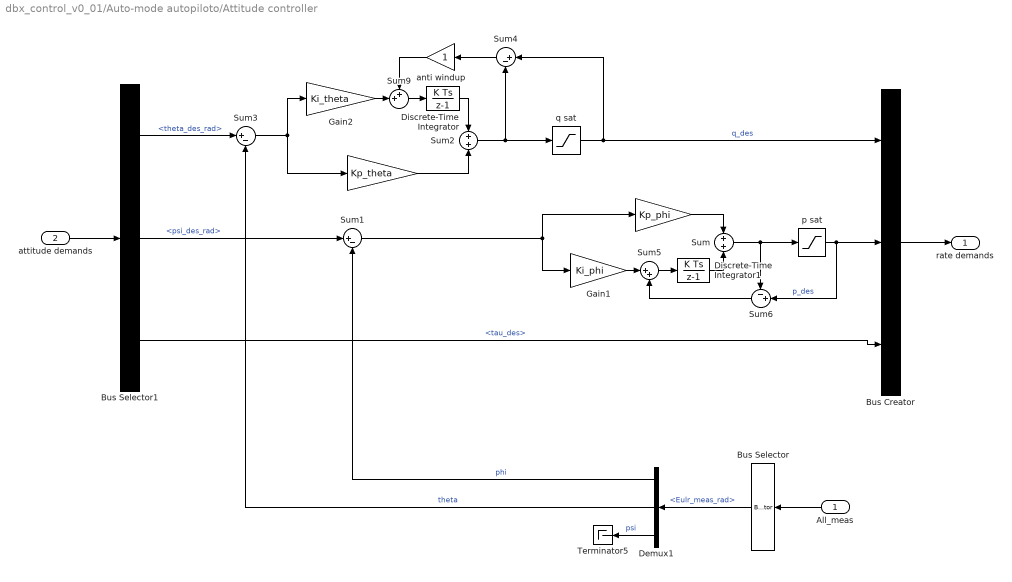
== system dbx_control_v0_01/Auto-mode autopiloto/Attitude controller ==
  All_meas : Inport
  attitude demands : Inport  Port=2
  " " : Gain  Gain=Kp_theta
  "  " : Gain  Gain=Kp_phi
  Bus Creator : BusCreator  Inputs=3
  Bus Selector : BusSelector  OutputSignals=Meas.Eulr_meas_rad
  Bus Selector1 : BusSelector  OutputSignals=theta_des_rad,psi_des_rad,tau_des
  Demux1 : Demux  Outputs=3
  Discrete-Time Integrator : DiscreteIntegrator  InitialConditionSetting=State (most efficient)  SampleTime=-1
  Discrete-Time Integrator1 : DiscreteIntegrator  InitialConditionSetting=State (most efficient)  SampleTime=-1
  Gain1 : Gain  Gain=Ki_phi
  Gain2 : Gain  Gain=Ki_theta
  Sum : Sum  Inputs=+|+
  Sum1 : Sum  Inputs=|+-
  Sum2 : Sum  Inputs=+|+
  Sum3 : Sum  Inputs=|+-
  Sum4 : Sum  Inputs=|+-
  Sum5 : Sum  Inputs=|++
  Sum6 : Sum  Inputs=-+|
  Sum9 : Sum  Inputs=++|
  Terminator5 : Terminator
  anti windup : Gain
  p sat : Saturate  UpperLimit=70*pi/180  LowerLimit=-70*pi/180  ZeroCross=off
  q sat : Saturate  UpperLimit=700*pi/180  LowerLimit=-700*pi/180  ZeroCross=off
  rate demands : Outport
  wires:
  Sum1/1 -> Gain1/1, "  "/1
  Bus Selector1/2 -> Sum1/1  "<psi_des_rad>"
  Sum3/1 -> Gain2/1, " "/1
  Discrete-Time Integrator/1 -> Sum2/1
  " "/1 -> Sum2/2
  Gain2/1 -> Sum9/2
  Sum9/1 -> Discrete-Time Integrator/1
  Sum2/1 -> q sat/1, Sum4/2
  q sat/1 -> Sum4/1, Bus Creator/1  "q_des"
  Sum4/1 -> anti windup/1
  anti windup/1 -> Sum9/1
  Discrete-Time Integrator1/1 -> Sum/2
  Sum/1 -> p sat/1, Sum6/1
  Bus Selector1/3 -> Bus Creator/3  "<tau_des>"
  Bus Selector1/1 -> Sum3/1  "<theta_des_rad>"
  "  "/1 -> Sum/1
  All_meas/1 -> Bus Selector/1
  Demux1/1 -> Sum1/2  "phi"
  Demux1/2 -> Sum3/2  "theta"
  Demux1/3 -> Terminator5/1  "psi"
  p sat/1 -> Bus Creator/2, Sum6/2  "p_des"
  Gain1/1 -> Sum5/1
  Sum5/1 -> Discrete-Time Integrator1/1
  Sum6/1 -> Sum5/2
  Bus Selector/1 -> Demux1/1  "<Eulr_meas_rad>"
  attitude demands/1 -> Bus Selector1/1
  Bus Creator/1 -> rate demands/1

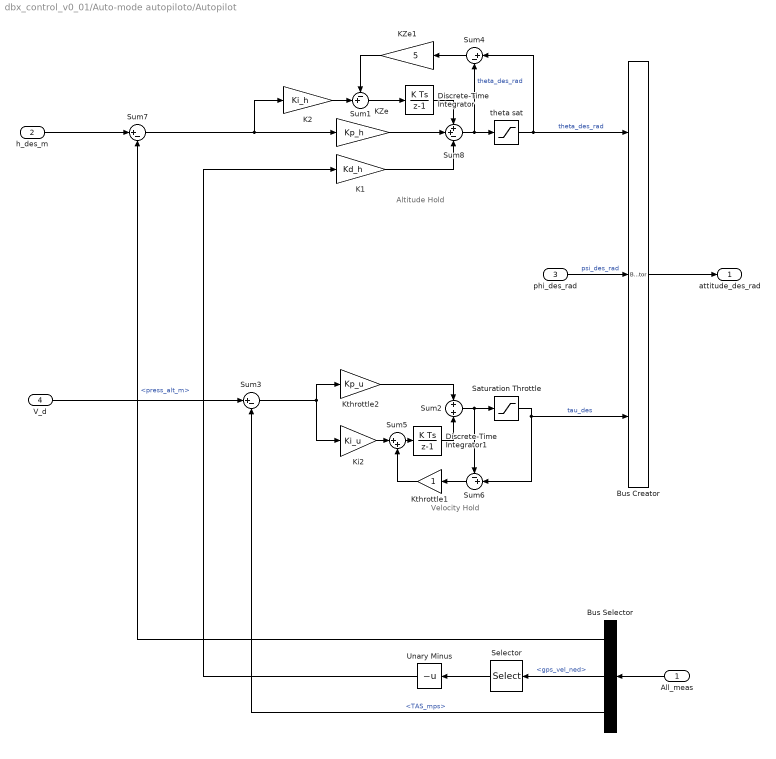
== system dbx_control_v0_01/Auto-mode autopiloto/Autopilot ==
  note: Velocity Hold
  note: Altitude Hold
  All_meas : Inport
  h_des_m : Inport  Port=2
  phi_des_rad : Inport  Port=3
  V_d : Inport  Port=4
  Bus Creator : BusCreator  Inputs=3
  Bus Selector : BusSelector  OutputSignals=Meas.press_alt_m,Meas.gps_vel_ned,Meas.TAS_mps
  Discrete-Time Integrator : DiscreteIntegrator  InitialCondition=Euler_0(2)  InitialConditionSetting=State (most efficient)  SampleTime=-1  LimitOutput=on  UpperSaturationLimit=0.3  LowerSaturationLimit=-0.3
  Discrete-Time Integrator1 : DiscreteIntegrator  InitialCondition=tau_1_0  InitialConditionSetting=State (most efficient)  SampleTime=-1  UpperSaturationLimit=0.3  LowerSaturationLimit=-0.3
  K1 : Gain  Gain=Kd_h
  K2 : Gain  Gain=Ki_h
  KZe : Gain  Gain=Kp_h
  KZe1 : Gain  Gain=5
  Ki2 : Gain  Gain=Ki_u
  Kthrottle1 : Gain
  Kthrottle2 : Gain  Gain=Kp_u
  Saturation Throttle : Saturate  UpperLimit=1  LowerLimit=0  ZeroCross=off
  Selector : Selector  InputPortWidth=3  Indices=3
  Sum1 : Sum  Inputs=-+|
  Sum2 : Sum
  Sum3 : Sum  Inputs=|+-
  Sum4 : Sum  Inputs=|+-
  Sum5 : Sum  Inputs=|++
  Sum6 : Sum  Inputs=-+|
  Sum7 : Sum  Inputs=|+-
  Sum8 : Sum  Inputs=++-
  Unary Minus : UnaryMinus
  theta sat : Saturate  UpperLimit=20*pi/180  LowerLimit=-10*pi/180  ZeroCross=off
  attitude_des_rad : Outport
  wires:
  Sum7/1 -> KZe/1, K2/1
  KZe/1 -> Sum8/2
  Sum1/1 -> Discrete-Time Integrator/1
  Discrete-Time Integrator/1 -> Sum8/1
  K1/1 -> Sum8/3
  Kthrottle2/1 -> Sum2/1
  Sum2/1 -> Saturation Throttle/1, Sum6/1
  Sum3/1 -> Kthrottle2/1, Ki2/1
  Saturation Throttle/1 -> Sum6/2, Bus Creator/3  "tau_des"
  Ki2/1 -> Sum5/1
  Sum5/1 -> Discrete-Time Integrator1/1
  Discrete-Time Integrator1/1 -> Sum2/2
  Sum6/1 -> Kthrottle1/1
  Kthrottle1/1 -> Sum5/2
  h_des_m/1 -> Sum7/1
  V_d/1 -> Sum3/1
  theta sat/1 -> Sum4/1, Bus Creator/1  "theta_des_rad"
  All_meas/1 -> Bus Selector/1
  Bus Creator/1 -> attitude_des_rad/1
  phi_des_rad/1 -> Bus Creator/2  "psi_des_rad"
  Bus Selector/1 -> Sum7/2  "<press_alt_m>"
  Bus Selector/2 -> Selector/1  "<gps_vel_ned>"
  Unary Minus/1 -> K1/1
  Bus Selector/3 -> Sum3/2  "<TAS_mps>"
  Selector/1 -> Unary Minus/1
  Sum4/1 -> KZe1/1
  Sum8/1 -> Sum4/2, theta sat/1  "theta_des_rad"
  K2/1 -> Sum1/2
  KZe1/1 -> Sum1/1

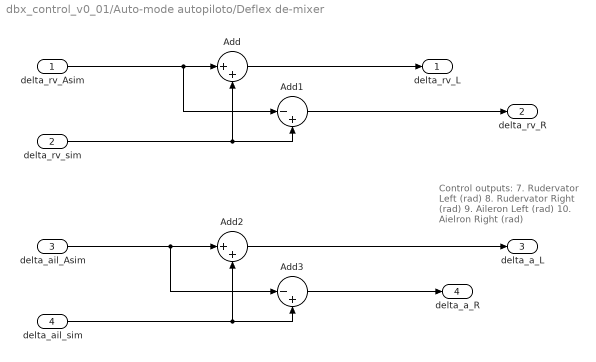
== system dbx_control_v0_01/Auto-mode autopiloto/Deflex de-mixer ==
  note: Control outputs:
      |
      | 7. Rudervator Left (rad)
      | 8. Rudervator Right (rad)
      | 9. Aileron Left (rad)
      | 10. Aielron Right (rad)
  delta_rv_Asim : Inport
  delta_rv_sim : Inport  Port=2
  delta_ail_Asim : Inport  Port=3
  delta_ail_sim : Inport  Port=4
  Add : Sum  Inputs=|++
  Add1 : Sum  Inputs=|-+
  Add2 : Sum  Inputs=|++
  Add3 : Sum  Inputs=|-+
  delta_rv_L : Outport
  delta_rv_R : Outport  Port=2
  delta_a_L : Outport  Port=3
  delta_a_R : Outport  Port=4
  wires:
  delta_rv_Asim/1 -> Add1/1, Add/1
  Add/1 -> delta_rv_L/1
  delta_rv_sim/1 -> Add1/2, Add/2
  Add1/1 -> delta_rv_R/1
  delta_ail_Asim/1 -> Add3/1, Add2/1
  Add2/1 -> delta_a_L/1
  delta_ail_sim/1 -> Add2/2, Add3/2
  Add3/1 -> delta_a_R/1

== system dbx_control_v0_01/Auto-mode autopiloto/Sample&Hold ==
  In1 : Inport
  Trigger : TriggerPort
  Out1 : Outport
  wires:
  In1/1 -> Out1/1

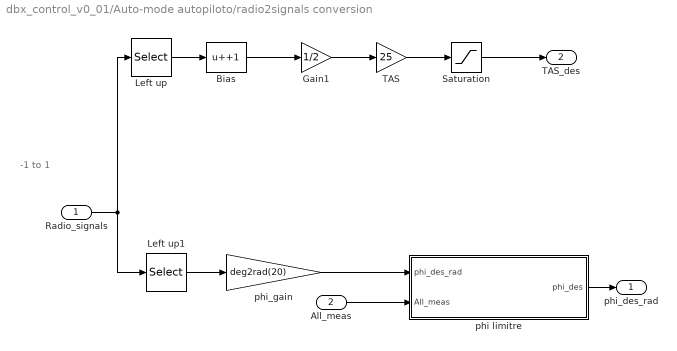
== system dbx_control_v0_01/Auto-mode autopiloto/radio2signals conversion ==
  note: -1 to 1
  Radio_signals : Inport
  All_meas : Inport  Port=2
  Bias : Bias  Bias=+1
  Gain1 : Gain  Gain=1/2
  Left up : Selector  InputPortWidth=4
  Left up1 : Selector  InputPortWidth=4  Indices=4
  Saturation : Saturate  UpperLimit=25  LowerLimit=15
  TAS : Gain  Gain=25
  phi limitre : Subsystem  TreatAsAtomicUnit=on
  phi_gain : Gain  Gain=deg2rad(20)
  phi_des_rad : Outport
  TAS_des : Outport  Port=2
  wires:
  Radio_signals/1 -> Left up/1, Left up1/1
  Bias/1 -> Gain1/1
  Left up/1 -> Bias/1
  Gain1/1 -> TAS/1
  TAS/1 -> Saturation/1
  Left up1/1 -> phi_gain/1
  All_meas/1 -> phi limitre/2(All_meas)
  phi_gain/1 -> phi limitre/1(phi_des_rad)
  Saturation/1 -> TAS_des/1
  phi limitre/1(phi_des) -> phi_des_rad/1

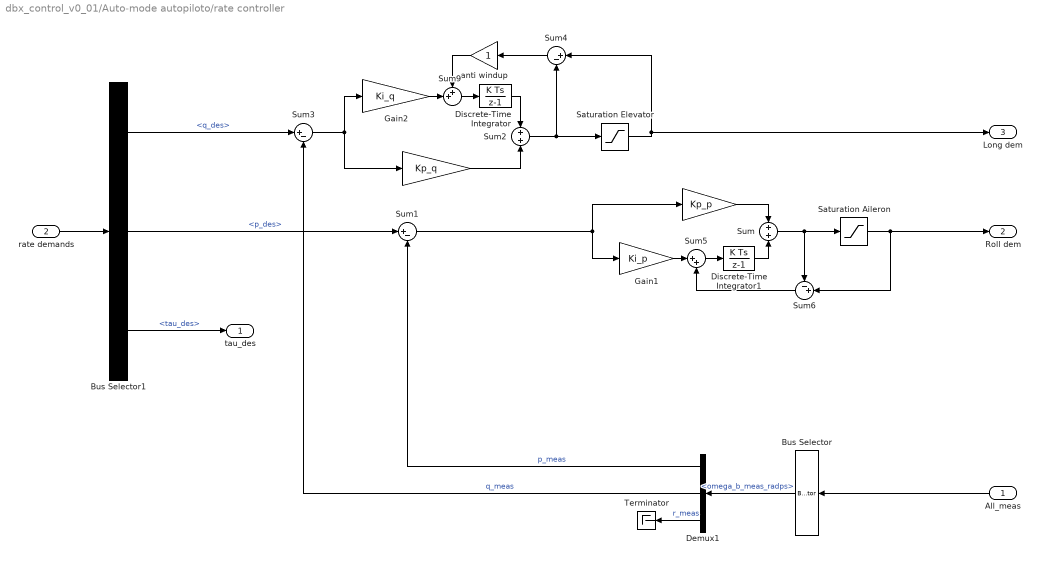
== system dbx_control_v0_01/Auto-mode autopiloto/rate controller ==
  All_meas : Inport
  rate demands : Inport  Port=2
  " " : Gain  Gain=Kp_q
  "  " : Gain  Gain=Kp_p
  Bus Selector : BusSelector  OutputSignals=Meas.omega_b_meas_radps
  Bus Selector1 : BusSelector  OutputSignals=q_des,p_des,tau_des
  Demux1 : Demux  Outputs=3
  Discrete-Time Integrator : DiscreteIntegrator  InitialCondition=delta_rv_sim_0 + Kp_q*Euler_0_2  InitialConditionSetting=State (most efficient)  SampleTime=-1
  Discrete-Time Integrator1 : DiscreteIntegrator  InitialCondition=delta_ail_Asim_0  InitialConditionSetting=State (most efficient)  SampleTime=-1
  Gain1 : Gain  Gain=Ki_p
  Gain2 : Gain  Gain=Ki_q
  Saturation Aileron : Saturate  UpperLimit=20*pi/180  LowerLimit=-20*pi/180  ZeroCross=off
  Saturation Elevator : Saturate  UpperLimit=20*pi/180  LowerLimit=-20*pi/180  ZeroCross=off
  Sum : Sum  Inputs=+|+
  Sum1 : Sum  Inputs=|+-
  Sum2 : Sum  Inputs=+|+
  Sum3 : Sum  Inputs=|+-
  Sum4 : Sum  Inputs=|+-
  Sum5 : Sum  Inputs=|++
  Sum6 : Sum  Inputs=-+|
  Sum9 : Sum  Inputs=++|
  Terminator : Terminator
  anti windup : Gain
  tau_des : Outport
  Roll dem : Outport  Port=2
  Long dem : Outport  Port=3
  wires:
  Bus Selector/1 -> Demux1/1  "<omega_b_meas_radps>"
  Sum6/1 -> Sum5/2
  Sum5/1 -> Discrete-Time Integrator1/1
  Gain1/1 -> Sum5/1
  Saturation Aileron/1 -> Roll dem/1, Sum6/2
  Demux1/2 -> Sum3/2  "q_meas"
  Demux1/1 -> Sum1/2  "p_meas"
  All_meas/1 -> Bus Selector/1
  "  "/1 -> Sum/1
  Bus Selector1/1 -> Sum3/1  "<q_des>"
  Bus Selector1/3 -> tau_des/1  "<tau_des>"
  Sum/1 -> Sum6/1, Saturation Aileron/1
  Discrete-Time Integrator1/1 -> Sum/2
  anti windup/1 -> Sum9/1
  Sum4/1 -> anti windup/1
  Saturation Elevator/1 -> Long dem/1, Sum4/1
  Sum2/1 -> Sum4/2, Saturation Elevator/1
  Sum9/1 -> Discrete-Time Integrator/1
  Gain2/1 -> Sum9/2
  " "/1 -> Sum2/2
  Discrete-Time Integrator/1 -> Sum2/1
  Sum3/1 -> " "/1, Gain2/1
  Bus Selector1/2 -> Sum1/1  "<p_des>"
  Sum1/1 -> Gain1/1, "  "/1
  rate demands/1 -> Bus Selector1/1
  Demux1/3 -> Terminator/1  "r_meas"

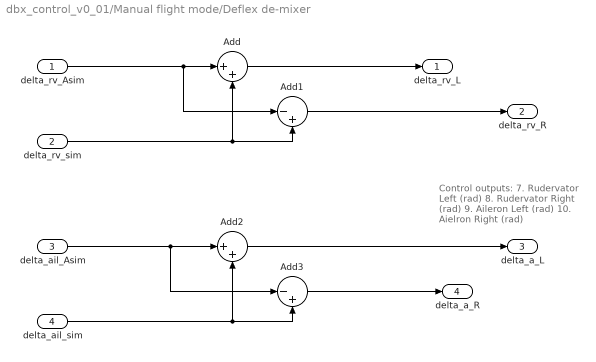
== system dbx_control_v0_01/Manual flight mode/Deflex de-mixer ==
  note: Control outputs:
      |
      | 7. Rudervator Left (rad)
      | 8. Rudervator Right (rad)
      | 9. Aileron Left (rad)
      | 10. Aielron Right (rad)
  delta_rv_Asim : Inport
  delta_rv_sim : Inport  Port=2
  delta_ail_Asim : Inport  Port=3
  delta_ail_sim : Inport  Port=4
  Add : Sum  Inputs=|++
  Add1 : Sum  Inputs=|-+
  Add2 : Sum  Inputs=|++
  Add3 : Sum  Inputs=|-+
  delta_rv_L : Outport
  delta_rv_R : Outport  Port=2
  delta_a_L : Outport  Port=3
  delta_a_R : Outport  Port=4
  wires:
  delta_rv_Asim/1 -> Add1/1, Add/1
  Add/1 -> delta_rv_L/1
  delta_rv_sim/1 -> Add1/2, Add/2
  Add1/1 -> delta_rv_R/1
  delta_ail_Asim/1 -> Add3/1, Add2/1
  Add2/1 -> delta_a_L/1
  delta_ail_sim/1 -> Add2/2, Add3/2
  Add3/1 -> delta_a_R/1

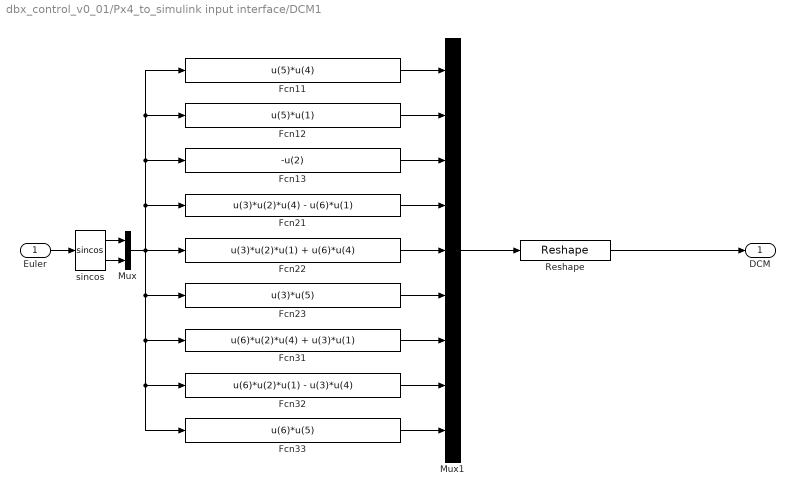
== system dbx_control_v0_01/Px4_to_simulink input interface/DCM1 ==
  Euler : Inport  PortDimensions=3
  Fcn11 : Fcn  Expr=u(5)*u(4)
  Fcn12 : Fcn  Expr=u(5)*u(1)
  Fcn13 : Fcn  Expr=-u(2)
  Fcn21 : Fcn  Expr=u(3)*u(2)*u(4) - u(6)*u(1)
  Fcn22 : Fcn  Expr=u(3)*u(2)*u(1) + u(6)*u(4)
  Fcn23 : Fcn  Expr=u(3)*u(5)
  Fcn31 : Fcn  Expr=u(6)*u(2)*u(4) + u(3)*u(1)
  Fcn32 : Fcn  Expr=u(6)*u(2)*u(1) - u(3)*u(4)
  Fcn33 : Fcn  Expr=u(6)*u(5)
  Mux : Mux  Inputs=2
  Mux1 : Mux  Inputs=9
  Reshape : Reshape  OutputDimensionality=Customize  OutputDimensions=[3,3]
  sincos : Trigonometry  Operator=sincos
  DCM : Outport  PortDimensions=[3,3]
  wires:
  Fcn33/1 -> Mux1/9
  Fcn32/1 -> Mux1/8
  Fcn23/1 -> Mux1/6
  Fcn22/1 -> Mux1/5
  Fcn31/1 -> Mux1/7
  Fcn21/1 -> Mux1/4
  Fcn13/1 -> Mux1/3
  Fcn12/1 -> Mux1/2
  Fcn11/1 -> Mux1/1
  Mux/1 -> Fcn22/1, Fcn23/1, Fcn31/1, Fcn33/1, Fcn32/1, Fcn21/1, Fcn13/1, Fcn12/1, Fcn11/1
  sincos/2 -> Mux/2
  sincos/1 -> Mux/1
  Reshape/1 -> DCM/1
  Euler/1 -> sincos/1
  Mux1/1 -> Reshape/1

== system dbx_control_v0_01/Auto-mode autopiloto/radio2signals conversion/phi limitre ==
  phi_des_rad : Inport
  All_meas : Inport  Port=2
  Bus Selector1 : BusSelector  OutputSignals=Meas.q_dyn_press
  C_L_max : Constant  Value=1.4
  Divide : Product  Inputs=*///
  Mass : Constant  Value=m
  Saturation Dynamic : simulink/Discontinuities/Saturation Dynamic  OutMin=[]  OutMax=[]  OutDataTypeStr=Inherit: Same as second input  OutDataType=fixdt(1, 16)  OutScaling=2^-10  DoSatur=off
  Sw : Constant  Value=S_w+0.15*1.38
  Trigonometric Function : Trigonometry  Operator=acos  OutputSignalType=real
  Unary Minus : UnaryMinus
  g : Gain  Gain=9.81
  phi_des : Outport
  wires:
  All_meas/1 -> Bus Selector1/1
  Unary Minus/1 -> Saturation Dynamic/3
  Saturation Dynamic/1 -> phi_des/1
  phi_des_rad/1 -> Saturation Dynamic/2
  Mass/1 -> g/1
  g/1 -> Divide/1
  Sw/1 -> Divide/2
  Bus Selector1/1 -> Divide/3  "<q_dyn_press>"
  C_L_max/1 -> Divide/4
  Divide/1 -> Trigonometric Function/1
  Trigonometric Function/1 -> Unary Minus/1, Saturation Dynamic/1

== matlab function dbx_control_v0_01/Px4_to_simulink input interface/MATLAB Function ==
  data: T_yaw output; yaw input
function T_yaw = Yaw_rotate(yaw)


T_yaw=[cos(yaw),    sin(yaw),   0;
        -sin(yaw),  cos(yaw),   0;
        0,      0,              1];
